simulink model "step_cmodel02_ol_2xPol"  (Simulink 7.9)
settings: Solver=ode45  StartTime=0.0  StopTime=10.0  RelTol=1e-9
values from neighbouring files (symbols this model uses):
  cwn = 2*xi*wn    (= 16)    [2xPol.m]    (also in cmodel_data.m = 22.5)
  initE = -1    [2xPol.m]    (also in cmodel_data.m = -0.0789832)
  kp = 1    [2xPol.m]
  T = 1/60    (= 0.0166666666667)    [cmodel_data.m]
  wn = 20    [2xPol.m]    (also in cmodel_data.m = 45)
settings Model: Creator=ex16  LastModifiedBy=ex16

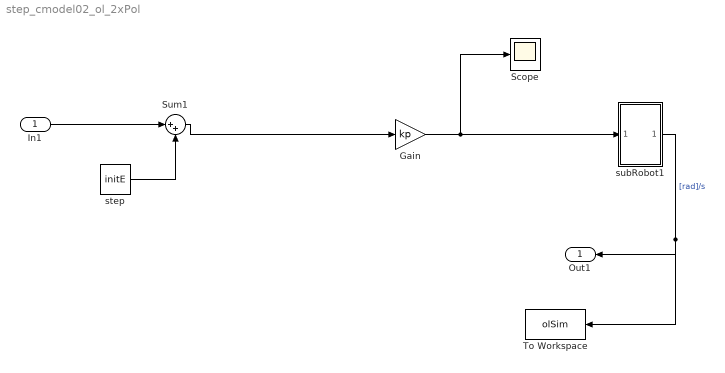
== system step_cmodel02_ol_2xPol ==
  In1 : Inport
  Gain : Gain  Gain=kp
  Scope : Scope
      settings: TimeRange=2  YMin=0  YMax=0.25
  Sum1 : Sum  Inputs=|++
  To Workspace : ToWorkspace  VariableName=olSim  SampleTime=-1  SaveFormat=Structure With Time
  step : Constant  Value=initE
  subRobot1 : Subsystem
  Out1 : Outport
  wires:
  In1/1 -> Sum1/1
  step/1 -> Sum1/2
  Sum1/1 -> Gain/1
  Gain/1 -> Scope/1, subRobot1/1(In1)
  subRobot1/1(Out1) -> To Workspace/1, Out1/1  "[rad]/s"

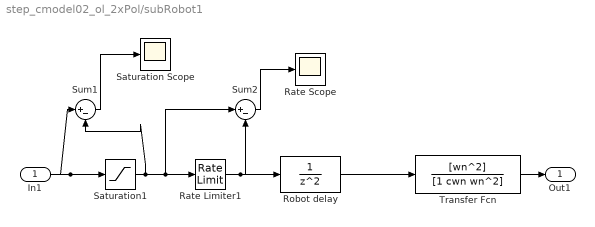
== system step_cmodel02_ol_2xPol/subRobot1 ==
  In1 : Inport
  Rate Limiter1 : RateLimiter  RisingSlewLimit=15  FallingSlewLimit=-15  SampleTimeMode=inherited
  Rate Scope : Scope
      settings: TimeRange=2  YMin=0  YMax=0.25  SaveName=ScopeData2
  Robot delay : DiscreteTransferFcn  Denominator=[1 0 0]  SampleTime=T
  Saturation Scope : Scope
  Saturation1 : Saturate  UpperLimit=3.2  LowerLimit=-3.2  SampleTime=T
  Sum1 : Sum  Inputs=|+-
  Sum2 : Sum  Inputs=|+-
  Transfer Fcn : TransferFcn  Numerator=[wn^2]  Denominator=[1 cwn wn^2]
  Out1 : Outport
  wires:
  Saturation1/1 -> Rate Limiter1/1, Sum2/1, Sum1/2
  Rate Limiter1/1 -> Robot delay/1, Sum2/2
  Sum2/1 -> Rate Scope/1
  In1/1 -> Saturation1/1, Sum1/1
  Sum1/1 -> Saturation Scope/1
  Transfer Fcn/1 -> Out1/1
  Robot delay/1 -> Transfer Fcn/1
